simulink model "test"  (R2020a)
settings: Solver=FixedStepAuto  StartTime=0.0  StopTime=10.0  FixedStep=1e-3  RelTol=1e-3  EnableMultiTasking=on
libraries: frdmk64flib x6, etargetslib x1
settings Model: ExtModeTrigDuration=5  Creator=Tim_G  LastModifiedBy=Tim_G
settings OptimizationCC: EnhancedBackFolding=on  PassReuseOutputArgsAs=Individual arguments  ZeroExternalMemoryAtStartup=off  ZeroInternalMemoryAtStartup=off  MaxStackSize=64  OptimizeBlockOrder=speed  DifferentSizesBufferReuse=on  OptimizationCustomize=off  EfficientTunableParamExpr=on
settings DebuggingCC: ParameterTunabilityLossMsg=error
settings HardwareCC: ProdBitPerPointer=32  ProdBitPerSizeT=32  ProdBitPerPtrDiffT=32  ProdLargestAtomicInteger=Long  ProdLargestAtomicFloat=Double  ProdWordSize=32  ProdHWDeviceType=ARM Compatible->ARM Cortex
settings SFSimCC: MATLABDynamicMemAlloc=off
settings RTWCC: SystemTargetFile=ert.tlc  HardwareBoard=NXP FRDM-K64F  TemplateMakefile=ert_default_tmf  Toolchain=GNU Tools for ARM Embedded Processors
settings CodeAppCC: ForceParamTrailComments=on  IgnoreCustomStorageClasses=off  OperatorAnnotations=on  SimulinkDataObjDesc=on  SFDataObjDesc=on  InsertBlockDesc=on

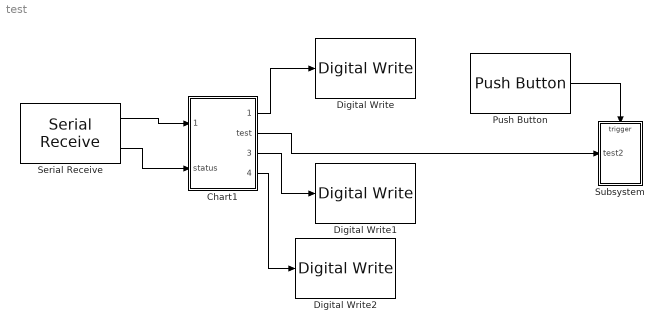
== system test ==
  Chart1 : Stateflow chart  TreatAsAtomicUnit=on
  Digital Write : frdmk64flib/Digital Write  Whichpin=RED_LED
  Digital Write1 : frdmk64flib/Digital Write  Whichpin=GREEN_LED
  Digital Write2 : frdmk64flib/Digital Write  Whichpin=BLUE_LED
  Push Button : frdmk64flib/Push Button  Whichswitch=SW2  SampleTime1=-1
  Serial Receive : frdmk64flib/Serial Receive  SCIModule=0  Baudrate=uint32(9600)  Parity=None  StopBits=1  HardwareFlowControl=None  ByteOrder=LittleEndian  DataType=uint8  DataLength=5  BlockingMode=off  OutputStatus=on  SampleTime=-1
  Subsystem : Subsystem
  wires:
  Push Button/1 -> Subsystem/Trigger
  Serial Receive/1 -> Chart1/1(rxdata)
  Serial Receive/2 -> Chart1/2(status)
  Chart1/1(R_LED) -> Digital Write/1
  Chart1/2(test) -> Subsystem/1(test2)
  Chart1/3(G_LED) -> Digital Write1/1
  Chart1/4(B_LED) -> Digital Write2/1

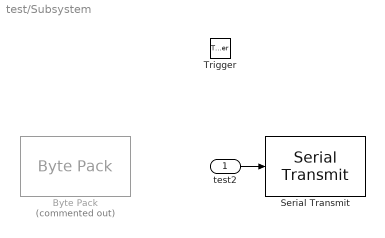
== system test/Subsystem ==
  test2 : Inport  OutDataTypeStr=uint8
  Trigger : TriggerPort  VariantControl=Variant  PortDimensions=1
  Byte Pack : etargetslib/Byte Pack  Commented=on  datatypes={'single'}  byteAlign=1
  Serial Transmit : frdmk64flib/Serial Transmit  SCIModule=0  Baudrate=uint32(9600)  Parity=None  StopBits=1  HardwareFlowControl=None  ByteOrder=LittleEndian  BlockingMode=on  OutputStatus=off
  wires:
  test2/1 -> Serial Transmit/1

== stateflow chart test/Chart1 ==
  state Receive1
    entry:
    test=data;
    G_LED=true;
  state Receive
    entry:
    test=data;
    R_LED=true;
  state Standby
    %Waiting for Data
    exit:
    data=rxdata;
  state Checksum
    entry:
    % compare checksum first
    % if checksum is valid, operate according to FnCode
    CHECKSUM=data(5);
    CHECKSUM_REAL=bitsxor(data(1:4));
  state Receive2
    entry:
    test=data;
    B_LED=true;
  Receive1 -> Standby
  (junction 17) -> Standby [order 4]
  Checksum -> Standby [order 2]
  (junction 17) -> Receive1 [order 2] : [data(2)==0x01]
  (default) -> Standby
  (junction 3) -> Standby [order 2]
  Checksum -> (junction 17) [order 1] : [CHECKSUM_REAL==CHECKSUM]
  Standby -> (junction 3) : [status==0]
  (junction 3) -> Checksum [order 1] : [rxdata(1)==hex2dec('55')]{R_LED=false;G_LED=false;B_LED=false}
  (junction 17) -> Receive [order 1] : [data(2)==0x00]
  (junction 17) -> Receive2 [order 3] : [data(2)==0x02]
  Receive -> Standby
  Receive2 -> Standby
  data: checksum function_output uint8 size=1; data_array function_input uint8; rxdata input uint8; status input; R_LED output; test output uint8; G_LED output; CHECKSUM_REAL local uint8; CHECKSUM local uint8; data local uint8; B_LED output
  function checksum=bitsxor(data_array):
    | function checksum=bitsxor(data_array)
    |     % calculate checksum
    |     % input: data_array is array of uint8 numbers
    |     % output: checksum (uint8) is bit-wise XOR of all uint8 data in the array
    |     checksum=data_array(1);
    |     for i=2:length(data_array)
    |         checksum = bitxor(checksum,data_array(i)); 
    |     end
    | end
